simulink model "practica5_ev3"  (R2016a)
settings: Solver=FixedStepAuto  StartTime=0.0  StopTime=60  FixedStep=0.032  RelTol=1e-3
libraries: legoev3lib x4
settings Model: ExtModeTrigDuration=2  Creator=jafma  LastModifiedBy=ruben
settings SolverCC: PositivePriorityOrder=on
settings OptimizationCC: MaxStackSize=64
settings HardwareCC: ProdBitPerPointer=32  ProdLargestAtomicInteger=Long  ProdWordSize=32  ProdHWDeviceType=ARM Compatible->ARM 9  UseEmbeddedCoderFeatures=off  UseSimulinkCoderFeatures=off
settings RTWCC: SystemTargetFile=ert.tlc  HardwareBoard=LEGO MINDSTORMS EV3  TLCOptions=-aInlineSetEventsForThisBaseRateFcn=TLC_FALSE -aSuppressMultiTaskScheduler=TLC_FALSE -aRateBasedStepFcn=0  TemplateMakefile=ert_default_tmf  GenerateReport=on  Toolchain=Sourcery G++ Lite v2009q3  LaunchReport=on
settings CodeAppCC: ForceParamTrailComments=on  OperatorAnnotations=on  MATLABSourceComments=on
settings ERTTargetCC: ERTCustomFileBanners=off  SupportContinuousTime=on  SupportNonInlinedSFcns=on  SupportVariableSizeSignals=on  ModelStepFunctionPrototypeControlCompliant=off

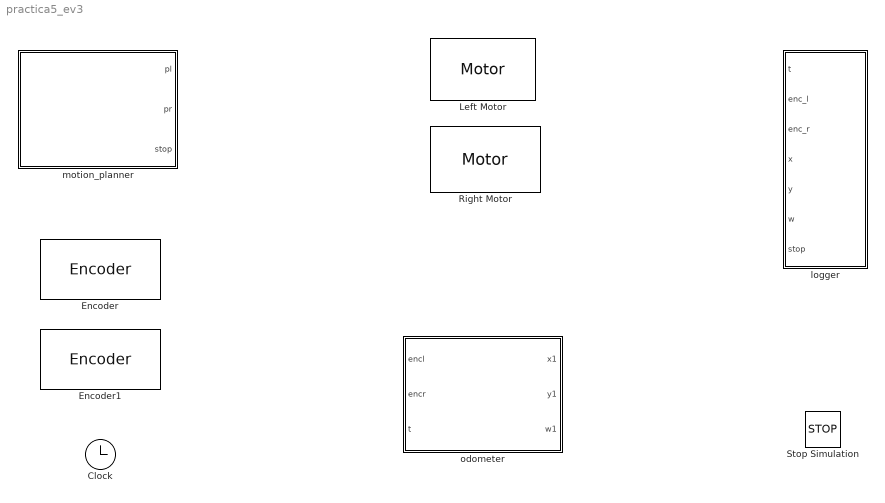
== system practica5_ev3 ==
  Clock : Clock
  Encoder : legoev3lib/Encoder  portNumber=B  opMode=No reset  sampleTime=0.032
  Encoder1 : legoev3lib/Encoder  portNumber=C  opMode=No reset  sampleTime=0.032
  Left Motor : legoev3lib/Motor  sportNumber=B  sstopAction=Brake
  Right Motor : legoev3lib/Motor  sportNumber=C  sstopAction=Brake
  Stop Simulation : Stop
  logger : MATLAB Function  TreatAsAtomicUnit=on
  motion_planner : MATLAB Function  TreatAsAtomicUnit=on
  odometer : MATLAB Function  TreatAsAtomicUnit=on

== matlab function practica5_ev3/motion_planner ==
  data: pl output; pr output; stop output
function [pl,pr,stop]  = motion_planner()

    stop = 0;
    
end

== matlab function practica5_ev3/odometer ==
  data: encl input; x1 output; y1 output; w1 output; encr input; t input
function [x1,y1,w1]  = odometer( encl, encr, t )

    time  = double(t);
    enc_l = double(encl);
    enc_r = double(encr);

    % define constants
    persistent D R;
    if( isempty(D) )
        D = 0.117;
        R = 0.027;
    end

    % define previous state 
    persistent x0 y0 w0 t0 prev_enc_l prev_enc_r;
    if( isempty(x0) )
        x0 = 0;
        y0 = 0;
        w0 = 0;
        t0 = time;
        prev_enc_l = enc_l;
        prev_enc_r = enc_r;
    end

end

== matlab function practica5_ev3/logger ==
  data: t input; enc_l input; enc_r input; x input; y input; w input; stop input
function logger(t,enc_l,enc_r,x,y,w,stop)
    %#codegen
    persistent myfile;
    if (isempty(myfile))
        myfile = fopen('/home/root/lms2012/prjs/mw/mylog.rdf','w');
    end
    if (myfile>=0)
         if (stop==1)
             fclose(myfile);
             myfile = -1;
         else
            fprintf(myfile,'%f\t%f\t%f\t%f\t%f\t%f\t\n',t,double(enc_l),double(enc_r),x,y,w);                
         end
    end
        
end
